simulink model "IPD_full"  (R2015b)
settings: Solver=VariableStepAuto  StartTime=0.0  StopTime=0.1  RelTol=1e-3
undefined symbols (not defined in the file): Jr, Kd, Ke, Ki, Kp, Kt, La, N, Ra, Tfv
settings Model: Creator=Erlingur  LastModifiedBy=Erlingur

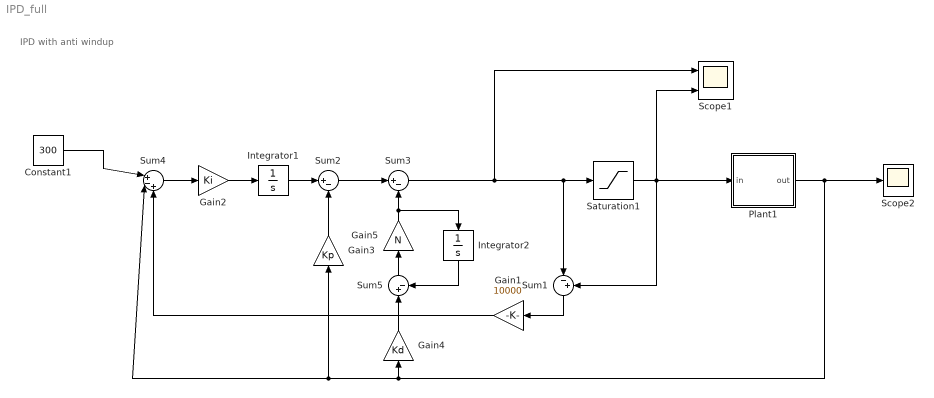
== system IPD_full ==
  note: IPD with anti windup
  Constant1 : Constant  Value=300
  Gain1 : Gain  Gain=10000
  Gain2 : Gain  Gain=Ki
  Gain3 : Gain  Gain=Kp
  Gain4 : Gain  Gain=Kd
  Gain5 : Gain  Gain=N
  Integrator1 : Integrator
  Integrator2 : Integrator
  Plant1 : Subsystem
  Saturation1 : Saturate  UpperLimit=15  LowerLimit=-15
  Scope1 : Scope  NumInputPorts=2
  Scope2 : Scope
  Sum1 : Sum  Inputs=|-+
  Sum2 : Sum  Inputs=|+-
  Sum3 : Sum  Inputs=|+-
  Sum4 : Sum  Inputs=|+-+
  Sum5 : Sum  Inputs=|+-
  wires:
  Sum5/1 -> Gain5/1
  Constant1/1 -> Sum4/1
  Sum2/1 -> Sum3/1
  Gain3/1 -> Sum2/2
  Sum4/1 -> Gain2/1
  Integrator1/1 -> Sum2/1
  Gain2/1 -> Integrator1/1
  Plant1/1(out) -> Scope2/1, Gain3/1, Sum4/2, Gain4/1
  Gain5/1 -> Integrator2/1, Sum3/2
  Gain4/1 -> Sum5/1
  Integrator2/1 -> Sum5/2
  Sum3/1 -> Scope1/1, Sum1/1, Saturation1/1
  Saturation1/1 -> Sum1/2, Scope1/2, Plant1/1(in)
  Sum1/1 -> Gain1/1
  Gain1/1 -> Sum4/3

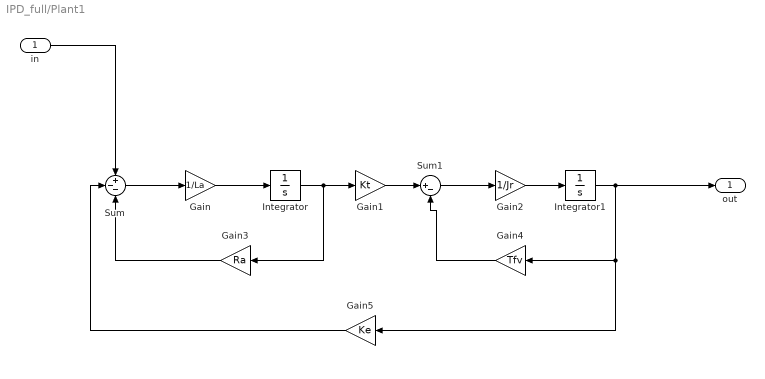
== system IPD_full/Plant1 ==
  in : Inport
  Gain : Gain  Gain=1/La
  Gain1 : Gain  Gain=Kt
  Gain2 : Gain  Gain=1/Jr
  Gain3 : Gain  Gain=Ra
  Gain4 : Gain  Gain=Tfv
  Gain5 : Gain  Gain=Ke
  Integrator : Integrator
  Integrator1 : Integrator
  Sum : Sum  Inputs=+--
  Sum1 : Sum  Inputs=|+-
  out : Outport
  wires:
  Sum1/1 -> Gain2/1
  Sum/1 -> Gain/1
  Integrator/1 -> Gain1/1, Gain3/1
  Gain/1 -> Integrator/1
  Gain5/1 -> Sum/2
  in/1 -> Sum/1
  Gain2/1 -> Integrator1/1
  Gain3/1 -> Sum/3
  Integrator1/1 -> out/1, Gain5/1, Gain4/1
  Gain4/1 -> Sum1/2
  Gain1/1 -> Sum1/1
